simulink model "LGS_allFaultsSelected"  (R2019b)
settings: Solver=FixedStepDiscrete  StartTime=0.0  StopTime=45.0  FixedStep=0.1  RelTol=1e-3
model workspace (MAT data in the model file):
  fipData : object (value not decoded)
  fipName : object (value not decoded)
  stepSize = 0.1
undefined symbols (not defined in the file): ActualSystemCondition, ExpectedSystemBehavior, FailureCondition, FailureConditionObserver, LibFailureCondition
libraries: LibFaultInjectionControls x190, commrandsrc3 x70, simulink x3
(part 6 of 41)

== system LGS_allFaultsSelected/Digital Part/Computing module1/GenericMonitoring1 ==
  In1 : Inport
  AND : Logic  Inputs=3  IconShape=distinctive  AllPortsSameDT=off  OutDataTypeStr=boolean
  Bus Selector : BusSelector  OutputSignals=signal1,signal2,signal3
  GenericMonitoring2 : Stateflow chart  TreatAsAtomicUnit=on
  Logical Operator1 : Logic  Operator=XOR  AllPortsSameDT=off  OutDataTypeStr=boolean
  Logical Operator2 : Logic  Operator=XOR  AllPortsSameDT=off  OutDataTypeStr=boolean
  Logical Operator3 : Logic  Operator=NOT  AllPortsSameDT=off  OutDataTypeStr=boolean
  Logical Operator4 : Logic  Operator=NOT  AllPortsSameDT=off  OutDataTypeStr=boolean
  Switch : Switch  Criteria=u2 > Threshold
  Switch1 : Switch  Criteria=u2 > Threshold
  Switch2 : Switch  Criteria=u2 > Threshold
  Signal : Outport  OutDataTypeStr=boolean
  Anomaly : Outport  Port=2  OutDataTypeStr=boolean
  wires:
  Bus Selector/1 -> GenericMonitoring2/1(Channel1), Logical Operator1/1, Switch1/1, Switch/1, AND/1  "<signal1>"
  Bus Selector/2 -> AND/2, GenericMonitoring2/2(Channel2), Logical Operator1/2, Logical Operator2/1, Switch2/1  "<signal2>"
  Bus Selector/3 -> AND/3, GenericMonitoring2/3(Channel3), Logical Operator2/2, Switch2/3  "<signal3>"
  In1/1 -> Bus Selector/1
  AND/1 -> Switch/2
  GenericMonitoring2/1(anomaly) -> Anomaly/1
  Switch/1 -> Signal/1
  Logical Operator4/1 -> Switch1/2
  Logical Operator2/1 -> Logical Operator3/1
  Switch2/1 -> Switch1/3
  Switch1/1 -> Switch/3
  Logical Operator3/1 -> Switch2/2
  Logical Operator1/1 -> Logical Operator4/1

== system LGS_allFaultsSelected/Digital Part/Computing module1/GenericMonitoring10 ==
  In1 : Inport
  AND : Logic  Inputs=3  IconShape=distinctive  AllPortsSameDT=off  OutDataTypeStr=boolean
  Bus Selector : BusSelector  OutputSignals=signal1,signal2,signal3
  GenericMonitoring2 : Stateflow chart  TreatAsAtomicUnit=on
  Logical Operator1 : Logic  Operator=XOR  AllPortsSameDT=off  OutDataTypeStr=boolean
  Logical Operator2 : Logic  Operator=XOR  AllPortsSameDT=off  OutDataTypeStr=boolean
  Logical Operator3 : Logic  Operator=NOT  AllPortsSameDT=off  OutDataTypeStr=boolean
  Logical Operator4 : Logic  Operator=NOT  AllPortsSameDT=off  OutDataTypeStr=boolean
  Switch : Switch  Criteria=u2 > Threshold
  Switch1 : Switch  Criteria=u2 > Threshold
  Switch2 : Switch  Criteria=u2 > Threshold
  Signal : Outport  OutDataTypeStr=boolean
  Anomaly : Outport  Port=2  OutDataTypeStr=boolean
  wires:
  Bus Selector/1 -> GenericMonitoring2/1(Channel1), Logical Operator1/1, Switch1/1, Switch/1, AND/1  "<signal1>"
  Bus Selector/2 -> AND/2, GenericMonitoring2/2(Channel2), Logical Operator1/2, Logical Operator2/1, Switch2/1  "<signal2>"
  Bus Selector/3 -> AND/3, GenericMonitoring2/3(Channel3), Logical Operator2/2, Switch2/3  "<signal3>"
  In1/1 -> Bus Selector/1
  AND/1 -> Switch/2
  GenericMonitoring2/1(anomaly) -> Anomaly/1
  Switch/1 -> Signal/1
  Logical Operator4/1 -> Switch1/2
  Logical Operator2/1 -> Logical Operator3/1
  Switch2/1 -> Switch1/3
  Switch1/1 -> Switch/3
  Logical Operator3/1 -> Switch2/2
  Logical Operator1/1 -> Logical Operator4/1

== system LGS_allFaultsSelected/Digital Part/Computing module1/GenericMonitoring11 ==
  In1 : Inport
  AND : Logic  Inputs=3  IconShape=distinctive  AllPortsSameDT=off  OutDataTypeStr=boolean
  Bus Selector : BusSelector  OutputSignals=signal1,signal2,signal3
  GenericMonitoring2 : Stateflow chart  TreatAsAtomicUnit=on
  Logical Operator1 : Logic  Operator=XOR  AllPortsSameDT=off  OutDataTypeStr=boolean
  Logical Operator2 : Logic  Operator=XOR  AllPortsSameDT=off  OutDataTypeStr=boolean
  Logical Operator3 : Logic  Operator=NOT  AllPortsSameDT=off  OutDataTypeStr=boolean
  Logical Operator4 : Logic  Operator=NOT  AllPortsSameDT=off  OutDataTypeStr=boolean
  Switch : Switch  Criteria=u2 > Threshold
  Switch1 : Switch  Criteria=u2 > Threshold
  Switch2 : Switch  Criteria=u2 > Threshold
  Signal : Outport  OutDataTypeStr=boolean
  Anomaly : Outport  Port=2  OutDataTypeStr=boolean
  wires:
  Bus Selector/1 -> GenericMonitoring2/1(Channel1), Logical Operator1/1, Switch1/1, Switch/1, AND/1  "<signal1>"
  Bus Selector/2 -> AND/2, GenericMonitoring2/2(Channel2), Logical Operator1/2, Logical Operator2/1, Switch2/1  "<signal2>"
  Bus Selector/3 -> AND/3, GenericMonitoring2/3(Channel3), Logical Operator2/2, Switch2/3  "<signal3>"
  In1/1 -> Bus Selector/1
  AND/1 -> Switch/2
  GenericMonitoring2/1(anomaly) -> Anomaly/1
  Switch/1 -> Signal/1
  Logical Operator4/1 -> Switch1/2
  Logical Operator2/1 -> Logical Operator3/1
  Switch2/1 -> Switch1/3
  Switch1/1 -> Switch/3
  Logical Operator3/1 -> Switch2/2
  Logical Operator1/1 -> Logical Operator4/1

== system LGS_allFaultsSelected/Digital Part/Computing module1/GenericMonitoring12 ==
  In1 : Inport
  AND : Logic  Inputs=3  IconShape=distinctive  AllPortsSameDT=off  OutDataTypeStr=boolean
  Bus Selector : BusSelector  OutputSignals=signal1,signal2,signal3
  GenericMonitoring2 : Stateflow chart  TreatAsAtomicUnit=on
  Logical Operator1 : Logic  Operator=XOR  AllPortsSameDT=off  OutDataTypeStr=boolean
  Logical Operator2 : Logic  Operator=XOR  AllPortsSameDT=off  OutDataTypeStr=boolean
  Logical Operator3 : Logic  Operator=NOT  AllPortsSameDT=off  OutDataTypeStr=boolean
  Logical Operator4 : Logic  Operator=NOT  AllPortsSameDT=off  OutDataTypeStr=boolean
  Switch : Switch  Criteria=u2 > Threshold
  Switch1 : Switch  Criteria=u2 > Threshold
  Switch2 : Switch  Criteria=u2 > Threshold
  Signal : Outport  OutDataTypeStr=boolean
  Anomaly : Outport  Port=2  OutDataTypeStr=boolean
  wires:
  Bus Selector/1 -> GenericMonitoring2/1(Channel1), Logical Operator1/1, Switch1/1, Switch/1, AND/1  "<signal1>"
  Bus Selector/2 -> AND/2, GenericMonitoring2/2(Channel2), Logical Operator1/2, Logical Operator2/1, Switch2/1  "<signal2>"
  Bus Selector/3 -> AND/3, GenericMonitoring2/3(Channel3), Logical Operator2/2, Switch2/3  "<signal3>"
  In1/1 -> Bus Selector/1
  AND/1 -> Switch/2
  GenericMonitoring2/1(anomaly) -> Anomaly/1
  Switch/1 -> Signal/1
  Logical Operator4/1 -> Switch1/2
  Logical Operator2/1 -> Logical Operator3/1
  Switch2/1 -> Switch1/3
  Switch1/1 -> Switch/3
  Logical Operator3/1 -> Switch2/2
  Logical Operator1/1 -> Logical Operator4/1

== system LGS_allFaultsSelected/Digital Part/Computing module1/GenericMonitoring13 ==
  In1 : Inport
  AND : Logic  Inputs=3  IconShape=distinctive  AllPortsSameDT=off  OutDataTypeStr=boolean
  Bus Selector : BusSelector  OutputSignals=signal1,signal2,signal3
  GenericMonitoring2 : Stateflow chart  TreatAsAtomicUnit=on
  Logical Operator1 : Logic  Operator=XOR  AllPortsSameDT=off  OutDataTypeStr=boolean
  Logical Operator2 : Logic  Operator=XOR  AllPortsSameDT=off  OutDataTypeStr=boolean
  Logical Operator3 : Logic  Operator=NOT  AllPortsSameDT=off  OutDataTypeStr=boolean
  Logical Operator4 : Logic  Operator=NOT  AllPortsSameDT=off  OutDataTypeStr=boolean
  Switch : Switch  Criteria=u2 > Threshold
  Switch1 : Switch  Criteria=u2 > Threshold
  Switch2 : Switch  Criteria=u2 > Threshold
  Signal : Outport  OutDataTypeStr=boolean
  Anomaly : Outport  Port=2  OutDataTypeStr=boolean
  wires:
  Bus Selector/1 -> GenericMonitoring2/1(Channel1), Logical Operator1/1, Switch1/1, Switch/1, AND/1  "<signal1>"
  Bus Selector/2 -> AND/2, GenericMonitoring2/2(Channel2), Logical Operator1/2, Logical Operator2/1, Switch2/1  "<signal2>"
  Bus Selector/3 -> AND/3, GenericMonitoring2/3(Channel3), Logical Operator2/2, Switch2/3  "<signal3>"
  In1/1 -> Bus Selector/1
  AND/1 -> Switch/2
  GenericMonitoring2/1(anomaly) -> Anomaly/1
  Switch/1 -> Signal/1
  Logical Operator4/1 -> Switch1/2
  Logical Operator2/1 -> Logical Operator3/1
  Switch2/1 -> Switch1/3
  Switch1/1 -> Switch/3
  Logical Operator3/1 -> Switch2/2
  Logical Operator1/1 -> Logical Operator4/1

== system LGS_allFaultsSelected/Digital Part/Computing module1/GenericMonitoring14 ==
  In1 : Inport
  AND : Logic  Inputs=3  IconShape=distinctive  AllPortsSameDT=off  OutDataTypeStr=boolean
  Bus Selector : BusSelector  OutputSignals=signal1,signal2,signal3
  GenericMonitoring2 : Stateflow chart  TreatAsAtomicUnit=on
  Logical Operator1 : Logic  Operator=XOR  AllPortsSameDT=off  OutDataTypeStr=boolean
  Logical Operator2 : Logic  Operator=XOR  AllPortsSameDT=off  OutDataTypeStr=boolean
  Logical Operator3 : Logic  Operator=NOT  AllPortsSameDT=off  OutDataTypeStr=boolean
  Logical Operator4 : Logic  Operator=NOT  AllPortsSameDT=off  OutDataTypeStr=boolean
  Switch : Switch  Criteria=u2 > Threshold
  Switch1 : Switch  Criteria=u2 > Threshold
  Switch2 : Switch  Criteria=u2 > Threshold
  Signal : Outport  OutDataTypeStr=boolean
  Anomaly : Outport  Port=2  OutDataTypeStr=boolean
  wires:
  Bus Selector/1 -> GenericMonitoring2/1(Channel1), Logical Operator1/1, Switch1/1, Switch/1, AND/1  "<signal1>"
  Bus Selector/2 -> AND/2, GenericMonitoring2/2(Channel2), Logical Operator1/2, Logical Operator2/1, Switch2/1  "<signal2>"
  Bus Selector/3 -> AND/3, GenericMonitoring2/3(Channel3), Logical Operator2/2, Switch2/3  "<signal3>"
  In1/1 -> Bus Selector/1
  AND/1 -> Switch/2
  GenericMonitoring2/1(anomaly) -> Anomaly/1
  Switch/1 -> Signal/1
  Logical Operator4/1 -> Switch1/2
  Logical Operator2/1 -> Logical Operator3/1
  Switch2/1 -> Switch1/3
  Switch1/1 -> Switch/3
  Logical Operator3/1 -> Switch2/2
  Logical Operator1/1 -> Logical Operator4/1

== system LGS_allFaultsSelected/Digital Part/Computing module1/GenericMonitoring15 ==
  In1 : Inport
  AND : Logic  Inputs=3  IconShape=distinctive  AllPortsSameDT=off  OutDataTypeStr=boolean
  Bus Selector : BusSelector  OutputSignals=signal1,signal2,signal3
  GenericMonitoring2 : Stateflow chart  TreatAsAtomicUnit=on
  Logical Operator1 : Logic  Operator=XOR  AllPortsSameDT=off  OutDataTypeStr=boolean
  Logical Operator2 : Logic  Operator=XOR  AllPortsSameDT=off  OutDataTypeStr=boolean
  Logical Operator3 : Logic  Operator=NOT  AllPortsSameDT=off  OutDataTypeStr=boolean
  Logical Operator4 : Logic  Operator=NOT  AllPortsSameDT=off  OutDataTypeStr=boolean
  Switch : Switch  Criteria=u2 > Threshold
  Switch1 : Switch  Criteria=u2 > Threshold
  Switch2 : Switch  Criteria=u2 > Threshold
  Signal : Outport  OutDataTypeStr=boolean
  Anomaly : Outport  Port=2  OutDataTypeStr=boolean
  wires:
  Bus Selector/1 -> GenericMonitoring2/1(Channel1), Logical Operator1/1, Switch1/1, Switch/1, AND/1  "<signal1>"
  Bus Selector/2 -> AND/2, GenericMonitoring2/2(Channel2), Logical Operator1/2, Logical Operator2/1, Switch2/1  "<signal2>"
  Bus Selector/3 -> AND/3, GenericMonitoring2/3(Channel3), Logical Operator2/2, Switch2/3  "<signal3>"
  In1/1 -> Bus Selector/1
  AND/1 -> Switch/2
  GenericMonitoring2/1(anomaly) -> Anomaly/1
  Switch/1 -> Signal/1
  Logical Operator4/1 -> Switch1/2
  Logical Operator2/1 -> Logical Operator3/1
  Switch2/1 -> Switch1/3
  Switch1/1 -> Switch/3
  Logical Operator3/1 -> Switch2/2
  Logical Operator1/1 -> Logical Operator4/1

== system LGS_allFaultsSelected/Digital Part/Computing module1/GenericMonitoring16 ==
  In1 : Inport
  AND : Logic  Inputs=3  IconShape=distinctive  AllPortsSameDT=off  OutDataTypeStr=boolean
  Bus Selector : BusSelector  OutputSignals=signal1,signal2,signal3
  GenericMonitoring2 : Stateflow chart  TreatAsAtomicUnit=on
  Logical Operator1 : Logic  Operator=XOR  AllPortsSameDT=off  OutDataTypeStr=boolean
  Logical Operator2 : Logic  Operator=XOR  AllPortsSameDT=off  OutDataTypeStr=boolean
  Logical Operator3 : Logic  Operator=NOT  AllPortsSameDT=off  OutDataTypeStr=boolean
  Logical Operator4 : Logic  Operator=NOT  AllPortsSameDT=off  OutDataTypeStr=boolean
  Switch : Switch  Criteria=u2 > Threshold
  Switch1 : Switch  Criteria=u2 > Threshold
  Switch2 : Switch  Criteria=u2 > Threshold
  Signal : Outport  OutDataTypeStr=boolean
  Anomaly : Outport  Port=2  OutDataTypeStr=boolean
  wires:
  Bus Selector/1 -> GenericMonitoring2/1(Channel1), Logical Operator1/1, Switch1/1, Switch/1, AND/1  "<signal1>"
  Bus Selector/2 -> AND/2, GenericMonitoring2/2(Channel2), Logical Operator1/2, Logical Operator2/1, Switch2/1  "<signal2>"
  Bus Selector/3 -> AND/3, GenericMonitoring2/3(Channel3), Logical Operator2/2, Switch2/3  "<signal3>"
  In1/1 -> Bus Selector/1
  AND/1 -> Switch/2
  GenericMonitoring2/1(anomaly) -> Anomaly/1
  Switch/1 -> Signal/1
  Logical Operator4/1 -> Switch1/2
  Logical Operator2/1 -> Logical Operator3/1
  Switch2/1 -> Switch1/3
  Switch1/1 -> Switch/3
  Logical Operator3/1 -> Switch2/2
  Logical Operator1/1 -> Logical Operator4/1

== system LGS_allFaultsSelected/Digital Part/Computing module1/GenericMonitoring17 ==
  In1 : Inport
  AND : Logic  Inputs=3  IconShape=distinctive  AllPortsSameDT=off  OutDataTypeStr=boolean
  Bus Selector : BusSelector  OutputSignals=signal1,signal2,signal3
  GenericMonitoring2 : Stateflow chart  TreatAsAtomicUnit=on
  Logical Operator1 : Logic  Operator=XOR  AllPortsSameDT=off  OutDataTypeStr=boolean
  Logical Operator2 : Logic  Operator=XOR  AllPortsSameDT=off  OutDataTypeStr=boolean
  Logical Operator3 : Logic  Operator=NOT  AllPortsSameDT=off  OutDataTypeStr=boolean
  Logical Operator4 : Logic  Operator=NOT  AllPortsSameDT=off  OutDataTypeStr=boolean
  Switch : Switch  Criteria=u2 > Threshold
  Switch1 : Switch  Criteria=u2 > Threshold
  Switch2 : Switch  Criteria=u2 > Threshold
  Signal : Outport  OutDataTypeStr=boolean
  Anomaly : Outport  Port=2  OutDataTypeStr=boolean
  wires:
  Bus Selector/1 -> GenericMonitoring2/1(Channel1), Logical Operator1/1, Switch1/1, Switch/1, AND/1  "<signal1>"
  Bus Selector/2 -> AND/2, GenericMonitoring2/2(Channel2), Logical Operator1/2, Logical Operator2/1, Switch2/1  "<signal2>"
  Bus Selector/3 -> AND/3, GenericMonitoring2/3(Channel3), Logical Operator2/2, Switch2/3  "<signal3>"
  In1/1 -> Bus Selector/1
  AND/1 -> Switch/2
  GenericMonitoring2/1(anomaly) -> Anomaly/1
  Switch/1 -> Signal/1
  Logical Operator4/1 -> Switch1/2
  Logical Operator2/1 -> Logical Operator3/1
  Switch2/1 -> Switch1/3
  Switch1/1 -> Switch/3
  Logical Operator3/1 -> Switch2/2
  Logical Operator1/1 -> Logical Operator4/1

== system LGS_allFaultsSelected/Digital Part/Computing module1/GenericMonitoring2 ==
  In1 : Inport
  AND : Logic  Inputs=3  IconShape=distinctive  AllPortsSameDT=off  OutDataTypeStr=boolean
  Bus Selector : BusSelector  OutputSignals=signal1,signal2,signal3
  GenericMonitoring2 : Stateflow chart  TreatAsAtomicUnit=on
  Logical Operator1 : Logic  Operator=XOR  AllPortsSameDT=off  OutDataTypeStr=boolean
  Logical Operator2 : Logic  Operator=XOR  AllPortsSameDT=off  OutDataTypeStr=boolean
  Logical Operator3 : Logic  Operator=NOT  AllPortsSameDT=off  OutDataTypeStr=boolean
  Logical Operator4 : Logic  Operator=NOT  AllPortsSameDT=off  OutDataTypeStr=boolean
  Switch : Switch  Criteria=u2 > Threshold
  Switch1 : Switch  Criteria=u2 > Threshold
  Switch2 : Switch  Criteria=u2 > Threshold
  Signal : Outport  OutDataTypeStr=boolean
  Anomaly : Outport  Port=2  OutDataTypeStr=boolean
  wires:
  Bus Selector/1 -> GenericMonitoring2/1(Channel1), Logical Operator1/1, Switch1/1, Switch/1, AND/1  "<signal1>"
  Bus Selector/2 -> AND/2, GenericMonitoring2/2(Channel2), Logical Operator1/2, Logical Operator2/1, Switch2/1  "<signal2>"
  Bus Selector/3 -> AND/3, GenericMonitoring2/3(Channel3), Logical Operator2/2, Switch2/3  "<signal3>"
  In1/1 -> Bus Selector/1
  AND/1 -> Switch/2
  GenericMonitoring2/1(anomaly) -> Anomaly/1
  Switch/1 -> Signal/1
  Logical Operator4/1 -> Switch1/2
  Logical Operator2/1 -> Logical Operator3/1
  Switch2/1 -> Switch1/3
  Switch1/1 -> Switch/3
  Logical Operator3/1 -> Switch2/2
  Logical Operator1/1 -> Logical Operator4/1

== system LGS_allFaultsSelected/Digital Part/Computing module1/GenericMonitoring3 ==
  In1 : Inport
  AND : Logic  Inputs=3  IconShape=distinctive  AllPortsSameDT=off  OutDataTypeStr=boolean
  Bus Selector : BusSelector  OutputSignals=signal1,signal2,signal3
  GenericMonitoring2 : Stateflow chart  TreatAsAtomicUnit=on
  Logical Operator1 : Logic  Operator=XOR  AllPortsSameDT=off  OutDataTypeStr=boolean
  Logical Operator2 : Logic  Operator=XOR  AllPortsSameDT=off  OutDataTypeStr=boolean
  Logical Operator3 : Logic  Operator=NOT  AllPortsSameDT=off  OutDataTypeStr=boolean
  Logical Operator4 : Logic  Operator=NOT  AllPortsSameDT=off  OutDataTypeStr=boolean
  Switch : Switch  Criteria=u2 > Threshold
  Switch1 : Switch  Criteria=u2 > Threshold
  Switch2 : Switch  Criteria=u2 > Threshold
  Signal : Outport  OutDataTypeStr=boolean
  Anomaly : Outport  Port=2  OutDataTypeStr=boolean
  wires:
  Bus Selector/1 -> GenericMonitoring2/1(Channel1), Logical Operator1/1, Switch1/1, Switch/1, AND/1  "<signal1>"
  Bus Selector/2 -> AND/2, GenericMonitoring2/2(Channel2), Logical Operator1/2, Logical Operator2/1, Switch2/1  "<signal2>"
  Bus Selector/3 -> AND/3, GenericMonitoring2/3(Channel3), Logical Operator2/2, Switch2/3  "<signal3>"
  In1/1 -> Bus Selector/1
  AND/1 -> Switch/2
  GenericMonitoring2/1(anomaly) -> Anomaly/1
  Switch/1 -> Signal/1
  Logical Operator4/1 -> Switch1/2
  Logical Operator2/1 -> Logical Operator3/1
  Switch2/1 -> Switch1/3
  Switch1/1 -> Switch/3
  Logical Operator3/1 -> Switch2/2
  Logical Operator1/1 -> Logical Operator4/1

== system LGS_allFaultsSelected/Digital Part/Computing module1/GenericMonitoring4 ==
  In1 : Inport
  AND : Logic  Inputs=3  IconShape=distinctive  AllPortsSameDT=off  OutDataTypeStr=boolean
  Bus Selector : BusSelector  OutputSignals=signal1,signal2,signal3
  GenericMonitoring2 : Stateflow chart  TreatAsAtomicUnit=on
  Logical Operator1 : Logic  Operator=XOR  AllPortsSameDT=off  OutDataTypeStr=boolean
  Logical Operator2 : Logic  Operator=XOR  AllPortsSameDT=off  OutDataTypeStr=boolean
  Logical Operator3 : Logic  Operator=NOT  AllPortsSameDT=off  OutDataTypeStr=boolean
  Logical Operator4 : Logic  Operator=NOT  AllPortsSameDT=off  OutDataTypeStr=boolean
  Switch : Switch  Criteria=u2 > Threshold
  Switch1 : Switch  Criteria=u2 > Threshold
  Switch2 : Switch  Criteria=u2 > Threshold
  Signal : Outport  OutDataTypeStr=boolean
  Anomaly : Outport  Port=2  OutDataTypeStr=boolean
  wires:
  Bus Selector/1 -> GenericMonitoring2/1(Channel1), Logical Operator1/1, Switch1/1, Switch/1, AND/1  "<signal1>"
  Bus Selector/2 -> AND/2, GenericMonitoring2/2(Channel2), Logical Operator1/2, Logical Operator2/1, Switch2/1  "<signal2>"
  Bus Selector/3 -> AND/3, GenericMonitoring2/3(Channel3), Logical Operator2/2, Switch2/3  "<signal3>"
  In1/1 -> Bus Selector/1
  AND/1 -> Switch/2
  GenericMonitoring2/1(anomaly) -> Anomaly/1
  Switch/1 -> Signal/1
  Logical Operator4/1 -> Switch1/2
  Logical Operator2/1 -> Logical Operator3/1
  Switch2/1 -> Switch1/3
  Switch1/1 -> Switch/3
  Logical Operator3/1 -> Switch2/2
  Logical Operator1/1 -> Logical Operator4/1

== system LGS_allFaultsSelected/Digital Part/Computing module1/GenericMonitoring5 ==
  In1 : Inport
  AND : Logic  Inputs=3  IconShape=distinctive  AllPortsSameDT=off  OutDataTypeStr=boolean
  Bus Selector : BusSelector  OutputSignals=signal1,signal2,signal3
  GenericMonitoring2 : Stateflow chart  TreatAsAtomicUnit=on
  Logical Operator1 : Logic  Operator=XOR  AllPortsSameDT=off  OutDataTypeStr=boolean
  Logical Operator2 : Logic  Operator=XOR  AllPortsSameDT=off  OutDataTypeStr=boolean
  Logical Operator3 : Logic  Operator=NOT  AllPortsSameDT=off  OutDataTypeStr=boolean
  Logical Operator4 : Logic  Operator=NOT  AllPortsSameDT=off  OutDataTypeStr=boolean
  Switch : Switch  Criteria=u2 > Threshold
  Switch1 : Switch  Criteria=u2 > Threshold
  Switch2 : Switch  Criteria=u2 > Threshold
  Signal : Outport  OutDataTypeStr=boolean
  Anomaly : Outport  Port=2  OutDataTypeStr=boolean
  wires:
  Bus Selector/1 -> GenericMonitoring2/1(Channel1), Logical Operator1/1, Switch1/1, Switch/1, AND/1  "<signal1>"
  Bus Selector/2 -> AND/2, GenericMonitoring2/2(Channel2), Logical Operator1/2, Logical Operator2/1, Switch2/1  "<signal2>"
  Bus Selector/3 -> AND/3, GenericMonitoring2/3(Channel3), Logical Operator2/2, Switch2/3  "<signal3>"
  In1/1 -> Bus Selector/1
  AND/1 -> Switch/2
  GenericMonitoring2/1(anomaly) -> Anomaly/1
  Switch/1 -> Signal/1
  Logical Operator4/1 -> Switch1/2
  Logical Operator2/1 -> Logical Operator3/1
  Switch2/1 -> Switch1/3
  Switch1/1 -> Switch/3
  Logical Operator3/1 -> Switch2/2
  Logical Operator1/1 -> Logical Operator4/1

== system LGS_allFaultsSelected/Digital Part/Computing module1/GenericMonitoring6 ==
  In1 : Inport
  AND : Logic  Inputs=3  IconShape=distinctive  AllPortsSameDT=off  OutDataTypeStr=boolean
  Bus Selector : BusSelector  OutputSignals=signal1,signal2,signal3
  GenericMonitoring2 : Stateflow chart  TreatAsAtomicUnit=on
  Logical Operator1 : Logic  Operator=XOR  AllPortsSameDT=off  OutDataTypeStr=boolean
  Logical Operator2 : Logic  Operator=XOR  AllPortsSameDT=off  OutDataTypeStr=boolean
  Logical Operator3 : Logic  Operator=NOT  AllPortsSameDT=off  OutDataTypeStr=boolean
  Logical Operator4 : Logic  Operator=NOT  AllPortsSameDT=off  OutDataTypeStr=boolean
  Switch : Switch  Criteria=u2 > Threshold
  Switch1 : Switch  Criteria=u2 > Threshold
  Switch2 : Switch  Criteria=u2 > Threshold
  Signal : Outport  OutDataTypeStr=boolean
  Anomaly : Outport  Port=2  OutDataTypeStr=boolean
  wires:
  Bus Selector/1 -> GenericMonitoring2/1(Channel1), Logical Operator1/1, Switch1/1, Switch/1, AND/1  "<signal1>"
  Bus Selector/2 -> AND/2, GenericMonitoring2/2(Channel2), Logical Operator1/2, Logical Operator2/1, Switch2/1  "<signal2>"
  Bus Selector/3 -> AND/3, GenericMonitoring2/3(Channel3), Logical Operator2/2, Switch2/3  "<signal3>"
  In1/1 -> Bus Selector/1
  AND/1 -> Switch/2
  GenericMonitoring2/1(anomaly) -> Anomaly/1
  Switch/1 -> Signal/1
  Logical Operator4/1 -> Switch1/2
  Logical Operator2/1 -> Logical Operator3/1
  Switch2/1 -> Switch1/3
  Switch1/1 -> Switch/3
  Logical Operator3/1 -> Switch2/2
  Logical Operator1/1 -> Logical Operator4/1

== system LGS_allFaultsSelected/Digital Part/Computing module1/GenericMonitoring7 ==
  In1 : Inport
  AND : Logic  Inputs=3  IconShape=distinctive  AllPortsSameDT=off  OutDataTypeStr=boolean
  Bus Selector : BusSelector  OutputSignals=signal1,signal2,signal3
  GenericMonitoring2 : Stateflow chart  TreatAsAtomicUnit=on
  Logical Operator1 : Logic  Operator=XOR  AllPortsSameDT=off  OutDataTypeStr=boolean
  Logical Operator2 : Logic  Operator=XOR  AllPortsSameDT=off  OutDataTypeStr=boolean
  Logical Operator3 : Logic  Operator=NOT  AllPortsSameDT=off  OutDataTypeStr=boolean
  Logical Operator4 : Logic  Operator=NOT  AllPortsSameDT=off  OutDataTypeStr=boolean
  Switch : Switch  Criteria=u2 > Threshold
  Switch1 : Switch  Criteria=u2 > Threshold
  Switch2 : Switch  Criteria=u2 > Threshold
  Signal : Outport  OutDataTypeStr=boolean
  Anomaly : Outport  Port=2  OutDataTypeStr=boolean
  wires:
  Bus Selector/1 -> GenericMonitoring2/1(Channel1), Logical Operator1/1, Switch1/1, Switch/1, AND/1  "<signal1>"
  Bus Selector/2 -> AND/2, GenericMonitoring2/2(Channel2), Logical Operator1/2, Logical Operator2/1, Switch2/1  "<signal2>"
  Bus Selector/3 -> AND/3, GenericMonitoring2/3(Channel3), Logical Operator2/2, Switch2/3  "<signal3>"
  In1/1 -> Bus Selector/1
  AND/1 -> Switch/2
  GenericMonitoring2/1(anomaly) -> Anomaly/1
  Switch/1 -> Signal/1
  Logical Operator4/1 -> Switch1/2
  Logical Operator2/1 -> Logical Operator3/1
  Switch2/1 -> Switch1/3
  Switch1/1 -> Switch/3
  Logical Operator3/1 -> Switch2/2
  Logical Operator1/1 -> Logical Operator4/1

== system LGS_allFaultsSelected/Digital Part/Computing module1/GenericMonitoring8 ==
  In1 : Inport
  AND : Logic  Inputs=3  IconShape=distinctive  AllPortsSameDT=off  OutDataTypeStr=boolean
  Bus Selector : BusSelector  OutputSignals=signal1,signal2,signal3
  GenericMonitoring2 : Stateflow chart  TreatAsAtomicUnit=on
  Logical Operator1 : Logic  Operator=XOR  AllPortsSameDT=off  OutDataTypeStr=boolean
  Logical Operator2 : Logic  Operator=XOR  AllPortsSameDT=off  OutDataTypeStr=boolean
  Logical Operator3 : Logic  Operator=NOT  AllPortsSameDT=off  OutDataTypeStr=boolean
  Logical Operator4 : Logic  Operator=NOT  AllPortsSameDT=off  OutDataTypeStr=boolean
  Switch : Switch  Criteria=u2 > Threshold
  Switch1 : Switch  Criteria=u2 > Threshold
  Switch2 : Switch  Criteria=u2 > Threshold
  Signal : Outport  OutDataTypeStr=boolean
  Anomaly : Outport  Port=2  OutDataTypeStr=boolean
  wires:
  Bus Selector/1 -> GenericMonitoring2/1(Channel1), Logical Operator1/1, Switch1/1, Switch/1, AND/1  "<signal1>"
  Bus Selector/2 -> AND/2, GenericMonitoring2/2(Channel2), Logical Operator1/2, Logical Operator2/1, Switch2/1  "<signal2>"
  Bus Selector/3 -> AND/3, GenericMonitoring2/3(Channel3), Logical Operator2/2, Switch2/3  "<signal3>"
  In1/1 -> Bus Selector/1
  AND/1 -> Switch/2
  GenericMonitoring2/1(anomaly) -> Anomaly/1
  Switch/1 -> Signal/1
  Logical Operator4/1 -> Switch1/2
  Logical Operator2/1 -> Logical Operator3/1
  Switch2/1 -> Switch1/3
  Switch1/1 -> Switch/3
  Logical Operator3/1 -> Switch2/2
  Logical Operator1/1 -> Logical Operator4/1

== system LGS_allFaultsSelected/Digital Part/Computing module1/GenericMonitoring9 ==
  In1 : Inport
  AND : Logic  Inputs=3  IconShape=distinctive  AllPortsSameDT=off  OutDataTypeStr=boolean
  Bus Selector : BusSelector  OutputSignals=signal1,signal2,signal3
  GenericMonitoring2 : Stateflow chart  TreatAsAtomicUnit=on
  Logical Operator1 : Logic  Operator=XOR  AllPortsSameDT=off  OutDataTypeStr=boolean
  Logical Operator2 : Logic  Operator=XOR  AllPortsSameDT=off  OutDataTypeStr=boolean
  Logical Operator3 : Logic  Operator=NOT  AllPortsSameDT=off  OutDataTypeStr=boolean
  Logical Operator4 : Logic  Operator=NOT  AllPortsSameDT=off  OutDataTypeStr=boolean
  Switch : Switch  Criteria=u2 > Threshold
  Switch1 : Switch  Criteria=u2 > Threshold
  Switch2 : Switch  Criteria=u2 > Threshold
  Signal : Outport  OutDataTypeStr=boolean
  Anomaly : Outport  Port=2  OutDataTypeStr=boolean
  wires:
  Bus Selector/1 -> GenericMonitoring2/1(Channel1), Logical Operator1/1, Switch1/1, Switch/1, AND/1  "<signal1>"
  Bus Selector/2 -> AND/2, GenericMonitoring2/2(Channel2), Logical Operator1/2, Logical Operator2/1, Switch2/1  "<signal2>"
  Bus Selector/3 -> AND/3, GenericMonitoring2/3(Channel3), Logical Operator2/2, Switch2/3  "<signal3>"
  In1/1 -> Bus Selector/1
  AND/1 -> Switch/2
  GenericMonitoring2/1(anomaly) -> Anomaly/1
  Switch/1 -> Signal/1
  Logical Operator4/1 -> Switch1/2
  Logical Operator2/1 -> Logical Operator3/1
  Switch2/1 -> Switch1/3
  Switch1/1 -> Switch/3
  Logical Operator3/1 -> Switch2/2
  Logical Operator1/1 -> Logical Operator4/1

== system LGS_allFaultsSelected/Digital Part/Computing module1/ReactToHandleChange ==
  In1 : Inport  OutDataTypeStr=boolean
  Delay1 : Delay  DelayLength=1  InitialCondition=0
  Delay2 : Delay  DelayLength=1  InitialCondition=0
  Logical Operator : Logic  AllPortsSameDT=off  OutDataTypeStr=boolean
  Logical Operator1 : Logic  Operator=NOT  AllPortsSameDT=off  OutDataTypeStr=boolean
  Logical Operator2 : Logic  AllPortsSameDT=off  OutDataTypeStr=boolean
  Logical Operator3 : Logic  Operator=NOT  AllPortsSameDT=off  OutDataTypeStr=boolean
  Extending : Outport  OutDataTypeStr=boolean
  Retracting : Outport  Port=2  OutDataTypeStr=boolean
  wires:
  In1/1 -> Delay2/1, Logical Operator2/2, Logical Operator1/1, Delay1/1
  Delay1/1 -> Logical Operator/1
  Logical Operator1/1 -> Logical Operator/2
  Logical Operator/1 -> Extending/1
  Logical Operator3/1 -> Logical Operator2/1
  Delay2/1 -> Logical Operator3/1
  Logical Operator2/1 -> Retracting/1

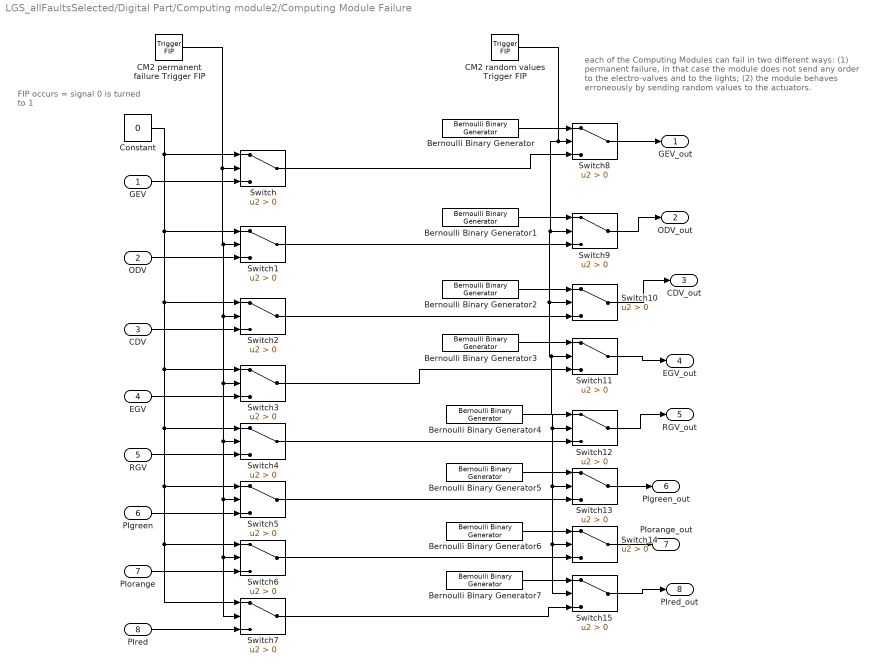
== system LGS_allFaultsSelected/Digital Part/Computing module2/Computing Module Failure ==
  note: FIP occurs = signal 0
      | is turned to 1
  note: each of the Computing Modules can fail in two different ways: (1) permanent failure, in that case the module does not send any order to the electro-valves and to the lights;
      | (2) the module behaves erroneously by sending random values to the actuators.
  GEV : Inport
  ODV : Inport  Port=2
  CDV : Inport  Port=3
  EGV : Inport  Port=4
  RGV : Inport  Port=5
  PIgreen : Inport  Port=6
  PIorange : Inport  Port=7
  PIred : Inport  Port=8
  Bernoulli Binary Generator{,1..7} (8 alike) : commrandsrc3/Bernoulli Binary Generator  ProbabilityOfZero=0.5  SeedSource=Auto  Seed=0  SampleTime=-1  SamplesPerFrame=1  OutputDataType=boolean  SimulateUsing=Interpreted execution
      settings: SourceProductName=Communications Toolbox
  CM2 permanent failure Trigger FIP : LibFaultInjectionControls/Trigger FIP  Active=on  MaintenanceTask=0  RiskTime=0  FailureRate=1.0E-4  isDSF=off  DSFjson=JSON
      settings: SourceProductName=Fault Injection Controls
  CM2 random values Trigger FIP : LibFaultInjectionControls/Trigger FIP  Active=on  MaintenanceTask=0  RiskTime=0  FailureRate=1.0E-4  isDSF=off  DSFjson=JSON
      settings: SourceProductName=Fault Injection Controls
  Constant : Constant  Value=0  OutDataTypeStr=boolean
  Switch{,1..15} (16 alike) : Switch  Criteria=u2 > Threshold
  GEV_out : Outport
  ODV_out : Outport  Port=2
  CDV_out : Outport  Port=3
  EGV_out : Outport  Port=4
  RGV_out : Outport  Port=5
  PIgreen_out : Outport  Port=6
  PIorange_out : Outport  Port=7
  PIred_out : Outport  Port=8
  wires:
  Constant/1 -> Switch4/1, Switch7/1, Switch6/1, Switch5/1, Switch3/1, Switch2/1, Switch1/1, Switch/1
  CM2 permanent failure Trigger FIP/1 -> Switch4/2, Switch7/2, Switch6/2, Switch5/2, Switch3/2, Switch2/2, Switch1/2, Switch/2
  GEV/1 -> Switch/3
  ODV/1 -> Switch1/3
  CDV/1 -> Switch2/3
  EGV/1 -> Switch3/3
  RGV/1 -> Switch4/3
  PIgreen/1 -> Switch5/3
  PIorange/1 -> Switch6/3
  PIred/1 -> Switch7/3
  Bernoulli Binary Generator/1 -> Switch8/1
  CM2 random values Trigger FIP/1 -> Switch15/2, Switch14/2, Switch13/2, Switch12/2, Switch11/2, Switch10/2, Switch9/2, Switch8/2
  Switch/1 -> Switch8/3
  Switch1/1 -> Switch9/3
  Switch2/1 -> Switch10/3
  Switch3/1 -> Switch11/3
  Switch4/1 -> Switch12/3
  Switch5/1 -> Switch13/3
  Switch6/1 -> Switch14/3
  Switch7/1 -> Switch15/3
  Switch8/1 -> GEV_out/1
  Switch9/1 -> ODV_out/1
  Switch10/1 -> CDV_out/1
  Switch11/1 -> EGV_out/1
  Switch12/1 -> RGV_out/1
  Switch13/1 -> PIgreen_out/1
  Switch14/1 -> PIorange_out/1
  Switch15/1 -> PIred_out/1
  Bernoulli Binary Generator1/1 -> Switch9/1
  Bernoulli Binary Generator2/1 -> Switch10/1
  Bernoulli Binary Generator3/1 -> Switch11/1
  Bernoulli Binary Generator4/1 -> Switch12/1
  Bernoulli Binary Generator5/1 -> Switch13/1
  Bernoulli Binary Generator6/1 -> Switch14/1
  Bernoulli Binary Generator7/1 -> Switch15/1

== system LGS_allFaultsSelected/Digital Part/Computing module2/GearsManeuvering ==
  not all doors locked closed : Inport
  not all gears locked extended : Inport  Port=2
  not all gears locked retracted : Inport  Port=3
  Logical Operator : Logic  Operator=OR  AllPortsSameDT=off  OutDataTypeStr=boolean
  Logical Operator1 : Logic  AllPortsSameDT=off  OutDataTypeStr=boolean
  maneuvering : Outport
  wires:
  not all doors locked closed/1 -> Logical Operator/1
  not all gears locked extended/1 -> Logical Operator1/1
  not all gears locked retracted/1 -> Logical Operator1/2
  Logical Operator/1 -> maneuvering/1
  Logical Operator1/1 -> Logical Operator/2

== system LGS_allFaultsSelected/Digital Part/Computing module2/GenericMonitoring ==
  In1 : Inport
  AND : Logic  Inputs=3  IconShape=distinctive  AllPortsSameDT=off  OutDataTypeStr=boolean
  Bus Selector : BusSelector  OutputSignals=signal1,signal2,signal3
  GenericMonitoring2 : Stateflow chart  TreatAsAtomicUnit=on
  Logical Operator1 : Logic  Operator=XOR  AllPortsSameDT=off  OutDataTypeStr=boolean
  Logical Operator2 : Logic  Operator=XOR  AllPortsSameDT=off  OutDataTypeStr=boolean
  Logical Operator3 : Logic  Operator=NOT  AllPortsSameDT=off  OutDataTypeStr=boolean
  Logical Operator4 : Logic  Operator=NOT  AllPortsSameDT=off  OutDataTypeStr=boolean
  Switch : Switch  Criteria=u2 > Threshold
  Switch1 : Switch  Criteria=u2 > Threshold
  Switch2 : Switch  Criteria=u2 > Threshold
  Signal : Outport  OutDataTypeStr=boolean
  Anomaly : Outport  Port=2  OutDataTypeStr=boolean
  wires:
  Bus Selector/1 -> GenericMonitoring2/1(Channel1), Logical Operator1/1, Switch1/1, Switch/1, AND/1  "<signal1>"
  Bus Selector/2 -> AND/2, GenericMonitoring2/2(Channel2), Logical Operator1/2, Logical Operator2/1, Switch2/1  "<signal2>"
  Bus Selector/3 -> AND/3, GenericMonitoring2/3(Channel3), Logical Operator2/2, Switch2/3  "<signal3>"
  In1/1 -> Bus Selector/1
  AND/1 -> Switch/2
  GenericMonitoring2/1(anomaly) -> Anomaly/1
  Switch/1 -> Signal/1
  Logical Operator4/1 -> Switch1/2
  Logical Operator2/1 -> Logical Operator3/1
  Switch2/1 -> Switch1/3
  Switch1/1 -> Switch/3
  Logical Operator3/1 -> Switch2/2
  Logical Operator1/1 -> Logical Operator4/1

== system LGS_allFaultsSelected/Digital Part/Computing module2/GenericMonitoring1 ==
  In1 : Inport
  AND : Logic  Inputs=3  IconShape=distinctive  AllPortsSameDT=off  OutDataTypeStr=boolean
  Bus Selector : BusSelector  OutputSignals=signal1,signal2,signal3
  GenericMonitoring2 : Stateflow chart  TreatAsAtomicUnit=on
  Logical Operator1 : Logic  Operator=XOR  AllPortsSameDT=off  OutDataTypeStr=boolean
  Logical Operator2 : Logic  Operator=XOR  AllPortsSameDT=off  OutDataTypeStr=boolean
  Logical Operator3 : Logic  Operator=NOT  AllPortsSameDT=off  OutDataTypeStr=boolean
  Logical Operator4 : Logic  Operator=NOT  AllPortsSameDT=off  OutDataTypeStr=boolean
  Switch : Switch  Criteria=u2 > Threshold
  Switch1 : Switch  Criteria=u2 > Threshold
  Switch2 : Switch  Criteria=u2 > Threshold
  Signal : Outport  OutDataTypeStr=boolean
  Anomaly : Outport  Port=2  OutDataTypeStr=boolean
  wires:
  Bus Selector/1 -> GenericMonitoring2/1(Channel1), Logical Operator1/1, Switch1/1, Switch/1, AND/1  "<signal1>"
  Bus Selector/2 -> AND/2, GenericMonitoring2/2(Channel2), Logical Operator1/2, Logical Operator2/1, Switch2/1  "<signal2>"
  Bus Selector/3 -> AND/3, GenericMonitoring2/3(Channel3), Logical Operator2/2, Switch2/3  "<signal3>"
  In1/1 -> Bus Selector/1
  AND/1 -> Switch/2
  GenericMonitoring2/1(anomaly) -> Anomaly/1
  Switch/1 -> Signal/1
  Logical Operator4/1 -> Switch1/2
  Logical Operator2/1 -> Logical Operator3/1
  Switch2/1 -> Switch1/3
  Switch1/1 -> Switch/3
  Logical Operator3/1 -> Switch2/2
  Logical Operator1/1 -> Logical Operator4/1

== system LGS_allFaultsSelected/Digital Part/Computing module2/GenericMonitoring10 ==
  In1 : Inport
  AND : Logic  Inputs=3  IconShape=distinctive  AllPortsSameDT=off  OutDataTypeStr=boolean
  Bus Selector : BusSelector  OutputSignals=signal1,signal2,signal3
  GenericMonitoring2 : Stateflow chart  TreatAsAtomicUnit=on
  Logical Operator1 : Logic  Operator=XOR  AllPortsSameDT=off  OutDataTypeStr=boolean
  Logical Operator2 : Logic  Operator=XOR  AllPortsSameDT=off  OutDataTypeStr=boolean
  Logical Operator3 : Logic  Operator=NOT  AllPortsSameDT=off  OutDataTypeStr=boolean
  Logical Operator4 : Logic  Operator=NOT  AllPortsSameDT=off  OutDataTypeStr=boolean
  Switch : Switch  Criteria=u2 > Threshold
  Switch1 : Switch  Criteria=u2 > Threshold
  Switch2 : Switch  Criteria=u2 > Threshold
  Signal : Outport  OutDataTypeStr=boolean
  Anomaly : Outport  Port=2  OutDataTypeStr=boolean
  wires:
  Bus Selector/1 -> GenericMonitoring2/1(Channel1), Logical Operator1/1, Switch1/1, Switch/1, AND/1  "<signal1>"
  Bus Selector/2 -> AND/2, GenericMonitoring2/2(Channel2), Logical Operator1/2, Logical Operator2/1, Switch2/1  "<signal2>"
  Bus Selector/3 -> AND/3, GenericMonitoring2/3(Channel3), Logical Operator2/2, Switch2/3  "<signal3>"
  In1/1 -> Bus Selector/1
  AND/1 -> Switch/2
  GenericMonitoring2/1(anomaly) -> Anomaly/1
  Switch/1 -> Signal/1
  Logical Operator4/1 -> Switch1/2
  Logical Operator2/1 -> Logical Operator3/1
  Switch2/1 -> Switch1/3
  Switch1/1 -> Switch/3
  Logical Operator3/1 -> Switch2/2
  Logical Operator1/1 -> Logical Operator4/1

== system LGS_allFaultsSelected/Digital Part/Computing module2/GenericMonitoring11 ==
  In1 : Inport
  AND : Logic  Inputs=3  IconShape=distinctive  AllPortsSameDT=off  OutDataTypeStr=boolean
  Bus Selector : BusSelector  OutputSignals=signal1,signal2,signal3
  GenericMonitoring2 : Stateflow chart  TreatAsAtomicUnit=on
  Logical Operator1 : Logic  Operator=XOR  AllPortsSameDT=off  OutDataTypeStr=boolean
  Logical Operator2 : Logic  Operator=XOR  AllPortsSameDT=off  OutDataTypeStr=boolean
  Logical Operator3 : Logic  Operator=NOT  AllPortsSameDT=off  OutDataTypeStr=boolean
  Logical Operator4 : Logic  Operator=NOT  AllPortsSameDT=off  OutDataTypeStr=boolean
  Switch : Switch  Criteria=u2 > Threshold
  Switch1 : Switch  Criteria=u2 > Threshold
  Switch2 : Switch  Criteria=u2 > Threshold
  Signal : Outport  OutDataTypeStr=boolean
  Anomaly : Outport  Port=2  OutDataTypeStr=boolean
  wires:
  Bus Selector/1 -> GenericMonitoring2/1(Channel1), Logical Operator1/1, Switch1/1, Switch/1, AND/1  "<signal1>"
  Bus Selector/2 -> AND/2, GenericMonitoring2/2(Channel2), Logical Operator1/2, Logical Operator2/1, Switch2/1  "<signal2>"
  Bus Selector/3 -> AND/3, GenericMonitoring2/3(Channel3), Logical Operator2/2, Switch2/3  "<signal3>"
  In1/1 -> Bus Selector/1
  AND/1 -> Switch/2
  GenericMonitoring2/1(anomaly) -> Anomaly/1
  Switch/1 -> Signal/1
  Logical Operator4/1 -> Switch1/2
  Logical Operator2/1 -> Logical Operator3/1
  Switch2/1 -> Switch1/3
  Switch1/1 -> Switch/3
  Logical Operator3/1 -> Switch2/2
  Logical Operator1/1 -> Logical Operator4/1

== system LGS_allFaultsSelected/Digital Part/Computing module2/GenericMonitoring12 ==
  In1 : Inport
  AND : Logic  Inputs=3  IconShape=distinctive  AllPortsSameDT=off  OutDataTypeStr=boolean
  Bus Selector : BusSelector  OutputSignals=signal1,signal2,signal3
  GenericMonitoring2 : Stateflow chart  TreatAsAtomicUnit=on
  Logical Operator1 : Logic  Operator=XOR  AllPortsSameDT=off  OutDataTypeStr=boolean
  Logical Operator2 : Logic  Operator=XOR  AllPortsSameDT=off  OutDataTypeStr=boolean
  Logical Operator3 : Logic  Operator=NOT  AllPortsSameDT=off  OutDataTypeStr=boolean
  Logical Operator4 : Logic  Operator=NOT  AllPortsSameDT=off  OutDataTypeStr=boolean
  Switch : Switch  Criteria=u2 > Threshold
  Switch1 : Switch  Criteria=u2 > Threshold
  Switch2 : Switch  Criteria=u2 > Threshold
  Signal : Outport  OutDataTypeStr=boolean
  Anomaly : Outport  Port=2  OutDataTypeStr=boolean
  wires:
  Bus Selector/1 -> GenericMonitoring2/1(Channel1), Logical Operator1/1, Switch1/1, Switch/1, AND/1  "<signal1>"
  Bus Selector/2 -> AND/2, GenericMonitoring2/2(Channel2), Logical Operator1/2, Logical Operator2/1, Switch2/1  "<signal2>"
  Bus Selector/3 -> AND/3, GenericMonitoring2/3(Channel3), Logical Operator2/2, Switch2/3  "<signal3>"
  In1/1 -> Bus Selector/1
  AND/1 -> Switch/2
  GenericMonitoring2/1(anomaly) -> Anomaly/1
  Switch/1 -> Signal/1
  Logical Operator4/1 -> Switch1/2
  Logical Operator2/1 -> Logical Operator3/1
  Switch2/1 -> Switch1/3
  Switch1/1 -> Switch/3
  Logical Operator3/1 -> Switch2/2
  Logical Operator1/1 -> Logical Operator4/1

== system LGS_allFaultsSelected/Digital Part/Computing module2/GenericMonitoring13 ==
  In1 : Inport
  AND : Logic  Inputs=3  IconShape=distinctive  AllPortsSameDT=off  OutDataTypeStr=boolean
  Bus Selector : BusSelector  OutputSignals=signal1,signal2,signal3
  GenericMonitoring2 : Stateflow chart  TreatAsAtomicUnit=on
  Logical Operator1 : Logic  Operator=XOR  AllPortsSameDT=off  OutDataTypeStr=boolean
  Logical Operator2 : Logic  Operator=XOR  AllPortsSameDT=off  OutDataTypeStr=boolean
  Logical Operator3 : Logic  Operator=NOT  AllPortsSameDT=off  OutDataTypeStr=boolean
  Logical Operator4 : Logic  Operator=NOT  AllPortsSameDT=off  OutDataTypeStr=boolean
  Switch : Switch  Criteria=u2 > Threshold
  Switch1 : Switch  Criteria=u2 > Threshold
  Switch2 : Switch  Criteria=u2 > Threshold
  Signal : Outport  OutDataTypeStr=boolean
  Anomaly : Outport  Port=2  OutDataTypeStr=boolean
  wires:
  Bus Selector/1 -> GenericMonitoring2/1(Channel1), Logical Operator1/1, Switch1/1, Switch/1, AND/1  "<signal1>"
  Bus Selector/2 -> AND/2, GenericMonitoring2/2(Channel2), Logical Operator1/2, Logical Operator2/1, Switch2/1  "<signal2>"
  Bus Selector/3 -> AND/3, GenericMonitoring2/3(Channel3), Logical Operator2/2, Switch2/3  "<signal3>"
  In1/1 -> Bus Selector/1
  AND/1 -> Switch/2
  GenericMonitoring2/1(anomaly) -> Anomaly/1
  Switch/1 -> Signal/1
  Logical Operator4/1 -> Switch1/2
  Logical Operator2/1 -> Logical Operator3/1
  Switch2/1 -> Switch1/3
  Switch1/1 -> Switch/3
  Logical Operator3/1 -> Switch2/2
  Logical Operator1/1 -> Logical Operator4/1

== system LGS_allFaultsSelected/Digital Part/Computing module2/GenericMonitoring14 ==
  In1 : Inport
  AND : Logic  Inputs=3  IconShape=distinctive  AllPortsSameDT=off  OutDataTypeStr=boolean
  Bus Selector : BusSelector  OutputSignals=signal1,signal2,signal3
  GenericMonitoring2 : Stateflow chart  TreatAsAtomicUnit=on
  Logical Operator1 : Logic  Operator=XOR  AllPortsSameDT=off  OutDataTypeStr=boolean
  Logical Operator2 : Logic  Operator=XOR  AllPortsSameDT=off  OutDataTypeStr=boolean
  Logical Operator3 : Logic  Operator=NOT  AllPortsSameDT=off  OutDataTypeStr=boolean
  Logical Operator4 : Logic  Operator=NOT  AllPortsSameDT=off  OutDataTypeStr=boolean
  Switch : Switch  Criteria=u2 > Threshold
  Switch1 : Switch  Criteria=u2 > Threshold
  Switch2 : Switch  Criteria=u2 > Threshold
  Signal : Outport  OutDataTypeStr=boolean
  Anomaly : Outport  Port=2  OutDataTypeStr=boolean
  wires:
  Bus Selector/1 -> GenericMonitoring2/1(Channel1), Logical Operator1/1, Switch1/1, Switch/1, AND/1  "<signal1>"
  Bus Selector/2 -> AND/2, GenericMonitoring2/2(Channel2), Logical Operator1/2, Logical Operator2/1, Switch2/1  "<signal2>"
  Bus Selector/3 -> AND/3, GenericMonitoring2/3(Channel3), Logical Operator2/2, Switch2/3  "<signal3>"
  In1/1 -> Bus Selector/1
  AND/1 -> Switch/2
  GenericMonitoring2/1(anomaly) -> Anomaly/1
  Switch/1 -> Signal/1
  Logical Operator4/1 -> Switch1/2
  Logical Operator2/1 -> Logical Operator3/1
  Switch2/1 -> Switch1/3
  Switch1/1 -> Switch/3
  Logical Operator3/1 -> Switch2/2
  Logical Operator1/1 -> Logical Operator4/1

== system LGS_allFaultsSelected/Digital Part/Computing module2/GenericMonitoring15 ==
  In1 : Inport
  AND : Logic  Inputs=3  IconShape=distinctive  AllPortsSameDT=off  OutDataTypeStr=boolean
  Bus Selector : BusSelector  OutputSignals=signal1,signal2,signal3
  GenericMonitoring2 : Stateflow chart  TreatAsAtomicUnit=on
  Logical Operator1 : Logic  Operator=XOR  AllPortsSameDT=off  OutDataTypeStr=boolean
  Logical Operator2 : Logic  Operator=XOR  AllPortsSameDT=off  OutDataTypeStr=boolean
  Logical Operator3 : Logic  Operator=NOT  AllPortsSameDT=off  OutDataTypeStr=boolean
  Logical Operator4 : Logic  Operator=NOT  AllPortsSameDT=off  OutDataTypeStr=boolean
  Switch : Switch  Criteria=u2 > Threshold
  Switch1 : Switch  Criteria=u2 > Threshold
  Switch2 : Switch  Criteria=u2 > Threshold
  Signal : Outport  OutDataTypeStr=boolean
  Anomaly : Outport  Port=2  OutDataTypeStr=boolean
  wires:
  Bus Selector/1 -> GenericMonitoring2/1(Channel1), Logical Operator1/1, Switch1/1, Switch/1, AND/1  "<signal1>"
  Bus Selector/2 -> AND/2, GenericMonitoring2/2(Channel2), Logical Operator1/2, Logical Operator2/1, Switch2/1  "<signal2>"
  Bus Selector/3 -> AND/3, GenericMonitoring2/3(Channel3), Logical Operator2/2, Switch2/3  "<signal3>"
  In1/1 -> Bus Selector/1
  AND/1 -> Switch/2
  GenericMonitoring2/1(anomaly) -> Anomaly/1
  Switch/1 -> Signal/1
  Logical Operator4/1 -> Switch1/2
  Logical Operator2/1 -> Logical Operator3/1
  Switch2/1 -> Switch1/3
  Switch1/1 -> Switch/3
  Logical Operator3/1 -> Switch2/2
  Logical Operator1/1 -> Logical Operator4/1

== system LGS_allFaultsSelected/Digital Part/Computing module2/GenericMonitoring16 ==
  In1 : Inport
  AND : Logic  Inputs=3  IconShape=distinctive  AllPortsSameDT=off  OutDataTypeStr=boolean
  Bus Selector : BusSelector  OutputSignals=signal1,signal2,signal3
  GenericMonitoring2 : Stateflow chart  TreatAsAtomicUnit=on
  Logical Operator1 : Logic  Operator=XOR  AllPortsSameDT=off  OutDataTypeStr=boolean
  Logical Operator2 : Logic  Operator=XOR  AllPortsSameDT=off  OutDataTypeStr=boolean
  Logical Operator3 : Logic  Operator=NOT  AllPortsSameDT=off  OutDataTypeStr=boolean
  Logical Operator4 : Logic  Operator=NOT  AllPortsSameDT=off  OutDataTypeStr=boolean
  Switch : Switch  Criteria=u2 > Threshold
  Switch1 : Switch  Criteria=u2 > Threshold
  Switch2 : Switch  Criteria=u2 > Threshold
  Signal : Outport  OutDataTypeStr=boolean
  Anomaly : Outport  Port=2  OutDataTypeStr=boolean
  wires:
  Bus Selector/1 -> GenericMonitoring2/1(Channel1), Logical Operator1/1, Switch1/1, Switch/1, AND/1  "<signal1>"
  Bus Selector/2 -> AND/2, GenericMonitoring2/2(Channel2), Logical Operator1/2, Logical Operator2/1, Switch2/1  "<signal2>"
  Bus Selector/3 -> AND/3, GenericMonitoring2/3(Channel3), Logical Operator2/2, Switch2/3  "<signal3>"
  In1/1 -> Bus Selector/1
  AND/1 -> Switch/2
  GenericMonitoring2/1(anomaly) -> Anomaly/1
  Switch/1 -> Signal/1
  Logical Operator4/1 -> Switch1/2
  Logical Operator2/1 -> Logical Operator3/1
  Switch2/1 -> Switch1/3
  Switch1/1 -> Switch/3
  Logical Operator3/1 -> Switch2/2
  Logical Operator1/1 -> Logical Operator4/1

== system LGS_allFaultsSelected/Digital Part/Computing module2/GenericMonitoring17 ==
  In1 : Inport
  AND : Logic  Inputs=3  IconShape=distinctive  AllPortsSameDT=off  OutDataTypeStr=boolean
  Bus Selector : BusSelector  OutputSignals=signal1,signal2,signal3
  GenericMonitoring2 : Stateflow chart  TreatAsAtomicUnit=on
  Logical Operator1 : Logic  Operator=XOR  AllPortsSameDT=off  OutDataTypeStr=boolean
  Logical Operator2 : Logic  Operator=XOR  AllPortsSameDT=off  OutDataTypeStr=boolean
  Logical Operator3 : Logic  Operator=NOT  AllPortsSameDT=off  OutDataTypeStr=boolean
  Logical Operator4 : Logic  Operator=NOT  AllPortsSameDT=off  OutDataTypeStr=boolean
  Switch : Switch  Criteria=u2 > Threshold
  Switch1 : Switch  Criteria=u2 > Threshold
  Switch2 : Switch  Criteria=u2 > Threshold
  Signal : Outport  OutDataTypeStr=boolean
  Anomaly : Outport  Port=2  OutDataTypeStr=boolean
  wires:
  Bus Selector/1 -> GenericMonitoring2/1(Channel1), Logical Operator1/1, Switch1/1, Switch/1, AND/1  "<signal1>"
  Bus Selector/2 -> AND/2, GenericMonitoring2/2(Channel2), Logical Operator1/2, Logical Operator2/1, Switch2/1  "<signal2>"
  Bus Selector/3 -> AND/3, GenericMonitoring2/3(Channel3), Logical Operator2/2, Switch2/3  "<signal3>"
  In1/1 -> Bus Selector/1
  AND/1 -> Switch/2
  GenericMonitoring2/1(anomaly) -> Anomaly/1
  Switch/1 -> Signal/1
  Logical Operator4/1 -> Switch1/2
  Logical Operator2/1 -> Logical Operator3/1
  Switch2/1 -> Switch1/3
  Switch1/1 -> Switch/3
  Logical Operator3/1 -> Switch2/2
  Logical Operator1/1 -> Logical Operator4/1

== system LGS_allFaultsSelected/Digital Part/Computing module2/GenericMonitoring2 ==
  In1 : Inport
  AND : Logic  Inputs=3  IconShape=distinctive  AllPortsSameDT=off  OutDataTypeStr=boolean
  Bus Selector : BusSelector  OutputSignals=signal1,signal2,signal3
  GenericMonitoring2 : Stateflow chart  TreatAsAtomicUnit=on
  Logical Operator1 : Logic  Operator=XOR  AllPortsSameDT=off  OutDataTypeStr=boolean
  Logical Operator2 : Logic  Operator=XOR  AllPortsSameDT=off  OutDataTypeStr=boolean
  Logical Operator3 : Logic  Operator=NOT  AllPortsSameDT=off  OutDataTypeStr=boolean
  Logical Operator4 : Logic  Operator=NOT  AllPortsSameDT=off  OutDataTypeStr=boolean
  Switch : Switch  Criteria=u2 > Threshold
  Switch1 : Switch  Criteria=u2 > Threshold
  Switch2 : Switch  Criteria=u2 > Threshold
  Signal : Outport  OutDataTypeStr=boolean
  Anomaly : Outport  Port=2  OutDataTypeStr=boolean
  wires:
  Bus Selector/1 -> GenericMonitoring2/1(Channel1), Logical Operator1/1, Switch1/1, Switch/1, AND/1  "<signal1>"
  Bus Selector/2 -> AND/2, GenericMonitoring2/2(Channel2), Logical Operator1/2, Logical Operator2/1, Switch2/1  "<signal2>"
  Bus Selector/3 -> AND/3, GenericMonitoring2/3(Channel3), Logical Operator2/2, Switch2/3  "<signal3>"
  In1/1 -> Bus Selector/1
  AND/1 -> Switch/2
  GenericMonitoring2/1(anomaly) -> Anomaly/1
  Switch/1 -> Signal/1
  Logical Operator4/1 -> Switch1/2
  Logical Operator2/1 -> Logical Operator3/1
  Switch2/1 -> Switch1/3
  Switch1/1 -> Switch/3
  Logical Operator3/1 -> Switch2/2
  Logical Operator1/1 -> Logical Operator4/1
